simulink model "Fixed_Wing_Model"  (R2023a)
settings: Solver=FixedStepAuto  StartTime=0.0  StopTime=inf  FixedStep=model_sampling_time  RelTol=1e-3
InitFcn:
  | run("Parameters.m")
values from neighbouring files (symbols this model uses):
  Alpha = params.Aerodynamics.Alpha    [aircraft_model.m]    (also in aircraft_params.mat = [-0.698131700798 -0.680678408278 -0.663225115758 -0.64577182; cost_straight_level.m = atan2(X(3), X(1)); create_table.m = deg2rad(-40:1:40)'; nonlinear_const.m = atan2(X(3), X(1)))
  Beta = params.Aerodynamics.Beta    [aircraft_model.m]    (also in aircraft_params.mat = [-0.349065850399 -0.261799387799 -0.174532925199 -0.08726646; create_table.m = deg2rad(-20:5:20)')
  CD_alpha_beta = [0.0544509195029 0.0530405310175 0.0517292718774 0.0505171420827 0.0494041416333 0.0483902705292 0.0474755287703 0.0466599163568 0.0459434332887 0.0453260795658 0.0448078551882 0.0443887601559 ... (729 elements, 81x9)]    [aircraft_params.mat]    (also in create_table.m = zeros(length(Alpha), length(Beta)))
  CD_alpha_dot = 0    [Parameters.m]    (also in aircraft_params.mat)
  CD_u = 0    [Parameters.m]    (also in aircraft_params.mat)
  CDda = [0 0 0 0 0 0 0 0 0 0 0 0 ... (1539 elements, 19x81)]    [aircraft_params.mat]    (also in create_table.m = zeros(length(da), length(Alpha)))
  CDde = [0 0 0 0 0 0 0 0 0 0 0 0 ... (1539 elements, 19x81)]    [aircraft_params.mat]    (also in create_table.m = zeros(length(de), length(Alpha)))
  CDdr = [0 0 0 0 0 0 0 0 0 0 0 0 ... (171 elements, 19x9)]    [aircraft_params.mat]    (also in create_table.m = zeros(length(dr), length(Beta)))
  CDp = [0.00874 0.009614 0.010488 0.011362 0.012236 0.01311 0.013984 0.014858 0.015732 0.016606 0.01748 0.018354 ... (81 elements, 81x1)]    [aircraft_params.mat]    (also in create_table.m = zeros(length(Alpha),1))
  CDq = [0 0 0 0 0 0 0 0 0 0 0 0 ... (81 elements, 81x1)]    [aircraft_params.mat]    (also in create_table.m = zeros(length(Alpha),1))
  CDr = [0 0 0 0 0 0 0 0 0 0 0 0 ... (81 elements, 81x1)]    [aircraft_params.mat]    (also in create_table.m = zeros(length(Alpha),1))
  chord = 0.1894    [Parameters.m]    (also in aircraft_model.m = params.chord; aircraft_params.mat)
  CL_alpha_beta = [-0.633037607685 -0.615603980908 -0.597456739131 -0.578694538839 -0.559464427591 -0.54002303701 -0.520877191922 -0.503102694522 -0.489045924609 -0.483759795494 -0.497410215644 -0.54697394645 ... (729 elements, 81x9)]    [aircraft_params.mat]    (also in create_table.m = zeros(length(Alpha), length(Beta)))
  Cl_alpha_beta = [0.00837758040957 0.00921533845053 0.0100530964915 0.0108908545324 0.0117286125734 0.0125663706144 0.0134041286553 0.0142418866963 0.0150796447372 0.0159174027782 0.0167551608191 0.0175929188601 ... (729 elements, 81x9)]    [aircraft_params.mat]    (also in create_table.m = zeros(length(Alpha), length(Beta)))
  CL_alpha_dot = 0    [Parameters.m]    (also in aircraft_params.mat)
  Cl_alpha_dot = 0    [Parameters.m]    (also in aircraft_params.mat)
  CL_u = 0    [Parameters.m]    (also in aircraft_params.mat)
  Cl_u = 0    [Parameters.m]    (also in aircraft_params.mat)
  CLda = [0 0 0 0 0 0 0 0 0 0 0 0 ... (1539 elements, 19x81)]    [aircraft_params.mat]    (also in create_table.m = zeros(length(da), length(Alpha)))
  Clda = [-0.0125663706144 -0.0111701072128 -0.00977384381117 -0.00837758040957 -0.00698131700798 -0.00558505360638 -0.00418879020479 -0.00279252680319 -0.0013962634016 0 0.0013962634016 0.00279252680319 ... (1539 elements, 19x81)]    [aircraft_params.mat]    (also in create_table.m = zeros(length(da), length(Alpha)))
  CLde = [0.0565486677646 0.0502654824574 0.0439822971503 0.0376991118431 0.0314159265359 0.0251327412287 0.0188495559215 0.0125663706144 0.00628318530718 0 -0.00628318530718 -0.0125663706144 ... (1539 elements, 19x81)]    [aircraft_params.mat]    (also in create_table.m = zeros(length(de), length(Alpha)))
  Clde = [0 0 0 0 0 0 0 0 0 0 0 0 ... (1539 elements, 19x81)]    [aircraft_params.mat]    (also in create_table.m = zeros(length(de), length(Alpha)))
  CLdr = [0 0 0 0 0 0 0 0 0 0 0 0 ... (171 elements, 19x9)]    [aircraft_params.mat]    (also in create_table.m = zeros(length(dr), length(Beta)))
  Cldr = [-0.0758694625842 -0.0674395222971 -0.0590095820099 -0.0505796417228 -0.0421497014357 -0.0337197611485 -0.0252898208614 -0.0168598805743 -0.00842994028713 0 0.00842994028713 0.0168598805743 ... (171 elements, 19x9)]    [aircraft_params.mat]    (also in create_table.m = zeros(length(dr), length(Beta)))
  CLp = [0 0 0 0 0 0 0 0 0 0 0 0 ... (81 elements, 81x1)]    [aircraft_params.mat]    (also in create_table.m = zeros(length(Alpha),1))
  Clp = [-0.052 -0.0572 -0.0624 -0.0676 -0.0728 -0.078 -0.0832 -0.0884 -0.0936 -0.0988 -0.104 -0.1092 ... (81 elements, 81x1)]    [aircraft_params.mat]    (also in create_table.m = zeros(length(Alpha),1))
  CLq = [0 0 0 0 0 0 0 0 0 0 0 0 ... (81 elements, 81x1)]    [aircraft_params.mat]    (also in create_table.m = zeros(length(Alpha),1))
  Clq = [0 0 0 0 0 0 0 0 0 0 0 0 ... (81 elements, 81x1)]    [aircraft_params.mat]    (also in create_table.m = zeros(length(Alpha),1))
  CLr = [0 0 0 0 0 0 0 0 0 0 0 0 ... (81 elements, 81x1)]    [aircraft_params.mat]    (also in create_table.m = zeros(length(Alpha),1))
  Clr = [0.028 0.0308 0.0336 0.0364 0.0392 0.042 0.0448 0.0476 0.0504 0.0532 0.056 0.0588 ... (81 elements, 81x1)]    [aircraft_params.mat]    (also in create_table.m = zeros(length(Alpha),1))
  Cm_alpha_beta = [0.220686842599 0.214585171534 0.208483500469 0.202381829404 0.196280158339 0.190178487274 0.184076816209 0.177975145144 0.171873474079 0.165771803014 0.159670131949 0.153568460884 ... (729 elements, 81x9)]    [aircraft_params.mat]    (also in create_table.m = zeros(length(Alpha), length(Beta)))
  Cm_alpha_dot = 0    [Parameters.m]    (also in aircraft_params.mat)
  Cm_u = 0    [Parameters.m]    (also in aircraft_params.mat)
  Cmda = [0 0 0 0 0 0 0 0 0 0 0 0 ... (1539 elements, 19x81)]    [aircraft_params.mat]    (also in create_table.m = zeros(length(da), length(Alpha)))
  Cmde = [0.0785398163397 0.0698131700798 0.0610865238198 0.0523598775598 0.0436332312999 0.0349065850399 0.0261799387799 0.0174532925199 0.00872664625997 0 -0.00872664625997 -0.0174532925199 ... (1539 elements, 19x81)]    [aircraft_params.mat]    (also in create_table.m = zeros(length(de), length(Alpha)))
  Cmdr = [0 0 0 0 0 0 0 0 0 0 0 0 ... (171 elements, 19x9)]    [aircraft_params.mat]    (also in create_table.m = zeros(length(dr), length(Beta)))
  Cmp = [0 0 0 0 0 0 0 0 0 0 0 0 ... (81 elements, 81x1)]    [aircraft_params.mat]    (also in create_table.m = zeros(length(Alpha),1))
  Cmq = [-0.72 -0.792 -0.864 -0.936 -1.008 -1.08 -1.152 -1.224 -1.296 -1.368 -1.44 -1.512 ... (81 elements, 81x1)]    [aircraft_params.mat]    (also in create_table.m = zeros(length(Alpha),1))
  Cmr = [0 0 0 0 0 0 0 0 0 0 0 0 ... (81 elements, 81x1)]    [aircraft_params.mat]    (also in create_table.m = zeros(length(Alpha),1))
  Cn_alpha_beta = [-0.0174532925199 -0.0191986217719 -0.0209439510239 -0.0226892802759 -0.0244346095279 -0.0261799387799 -0.0279252680319 -0.0296705972839 -0.0314159265359 -0.0331612557879 -0.0349065850399 -0.0366519142919 ... (729 elements, 81x9)]    [aircraft_params.mat]    (also in create_table.m = zeros(length(Alpha), length(Beta)))
  Cn_alpha_dot = 0    [Parameters.m]    (also in aircraft_params.mat)
  Cn_u = 0    [Parameters.m]    (also in aircraft_params.mat)
  Cnda = [-0.00942477796077 -0.00837758040957 -0.00733038285838 -0.00628318530718 -0.00523598775598 -0.00418879020479 -0.00314159265359 -0.00209439510239 -0.0010471975512 0 0.0010471975512 0.00209439510239 ... (1539 elements, 19x81)]    [aircraft_params.mat]    (also in create_table.m = zeros(length(da), length(Alpha)))
  Cnde = [0 0 0 0 0 0 0 0 0 0 0 0 ... (1539 elements, 19x81)]    [aircraft_params.mat]    (also in create_table.m = zeros(length(de), length(Alpha)))
  Cndr = [0.0231221219304 0.0205529972715 0.0179838726125 0.0154147479536 0.0128456232947 0.0102764986357 0.00770737397681 0.00513824931787 0.00256912465894 0 -0.00256912465894 -0.00513824931787 ... (171 elements, 19x9)]    [aircraft_params.mat]    (also in create_table.m = zeros(length(dr), length(Beta)))
  Cnp = [0.0044 0.00484 0.00528 0.00572 0.00616 0.0066 0.00704 0.00748 0.00792 0.00836 0.0088 0.00924 ... (81 elements, 81x1)]    [aircraft_params.mat]    (also in create_table.m = zeros(length(Alpha),1))
  Cnq = [0 0 0 0 0 0 0 0 0 0 0 0 ... (81 elements, 81x1)]    [aircraft_params.mat]    (also in create_table.m = zeros(length(Alpha),1))
  Cnr = [-0.07 -0.077 -0.084 -0.091 -0.098 -0.105 -0.112 -0.119 -0.126 -0.133 -0.14 -0.147 ... (81 elements, 81x1)]    [aircraft_params.mat]    (also in create_table.m = zeros(length(Alpha),1))
  CY_alpha_beta = [0.0684169066782 0.075258597346 0.0821002880138 0.0889419786816 0.0957836693494 0.102625360017 0.109467050685 0.116308741353 0.123150432021 0.129992122689 0.136833813356 0.143675504024 ... (729 elements, 81x9)]    [aircraft_params.mat]    (also in create_table.m = zeros(length(Alpha), length(Beta)))
  CY_alpha_dot = 0    [Parameters.m]    (also in aircraft_params.mat)
  CY_u = 0    [Parameters.m]    (also in aircraft_params.mat)
  CYda = [0 0 0 0 0 0 0 0 0 0 0 0 ... (1539 elements, 19x81)]    [aircraft_params.mat]    (also in create_table.m = zeros(length(da), length(Alpha)))
  CYde = [0 0 0 0 0 0 0 0 0 0 0 0 ... (1539 elements, 19x81)]    [aircraft_params.mat]    (also in create_table.m = zeros(length(de), length(Alpha)))
  CYdr = [0.122836272755 0.109187798005 0.0955393232542 0.0818908485036 0.068242373753 0.0545938990024 0.0409454242518 0.0272969495012 0.0136484747506 0 -0.0136484747506 -0.0272969495012 ... (171 elements, 19x9)]    [aircraft_params.mat]    (also in create_table.m = zeros(length(dr), length(Beta)))
  CYp = [0 0 0 0 0 0 0 0 0 0 0 0 ... (81 elements, 81x1)]    [aircraft_params.mat]    (also in create_table.m = zeros(length(Alpha),1))
  CYq = [0 0 0 0 0 0 0 0 0 0 0 0 ... (81 elements, 81x1)]    [aircraft_params.mat]    (also in create_table.m = zeros(length(Alpha),1))
  CYr = [0 0 0 0 0 0 0 0 0 0 0 0 ... (81 elements, 81x1)]    [aircraft_params.mat]    (also in create_table.m = zeros(length(Alpha),1))
  D = zeros(size(B_long))    [Linearized_Model.m]    (also in linear_models.mat = [0 0 0 0 0 0 0 0 0 0 0 0 ... (16 elements, 4x4)])
  da = params.Aerodynamics.da    [aircraft_model.m]    (also in aircraft_params.mat = [-0.785398163397 -0.698131700798 -0.610865238198 -0.52359877; create_table.m = deg2rad(-45:5:45))
  da_lim = deg2rad(45)    [Parameters.m]    (also in aircraft_model.m = params.da_lim; aircraft_params.mat = 0.785398163397)
  de_lim = deg2rad(45)    [Parameters.m]    (also in aircraft_model.m = params.de_lim; aircraft_params.mat = 0.785398163397)
  dr = params.Aerodynamics.dr    [aircraft_model.m]    (also in aircraft_params.mat = [-0.785398163397 -0.698131700798 -0.610865238198 -0.52359877; create_table.m = deg2rad(-45:5:45))
  dr_lim = deg2rad(45)    [Parameters.m]    (also in aircraft_model.m = params.dr_lim; aircraft_params.mat = 0.785398163397)
  dth_lim = 100    [Parameters.m]    (also in aircraft_model.m = params.dth_lim; aircraft_params.mat)
  h_ref = 0    [Parameters.m]    (also in aircraft_params.mat)
  Inertia_Tensor = [Jx -Jxy -Jxz ... (first row only)    [Parameters.m]    (also in aircraft_model.m; aircraft_params.mat = [0.8244  0  -0.1204; 0  1.135  0; -0.1204  0  1.759])
  lat_ref_deg = 40    [Parameters.m]    (also in aircraft_params.mat)
  long_ref_deg = 20    [Parameters.m]    (also in aircraft_params.mat)
  mass = 13.5    [Parameters.m]    (also in aircraft_model.m = params.mass; aircraft_params.mat)
  Motor =     [aircraft_params.mat]
  pqr_initial = [0; 0; 0]    [Parameters.m]    (also in aircraft_params.mat = [0 0 0])
  quat_initial = eul2quat(euler_initial')    [Parameters.m]    (also in aircraft_params.mat = [1 0 0 0])
  rho_msl = 1.225    [Parameters.m]    (also in aircraft_model.m = params.rho_msl; aircraft_params.mat)
  S = 2.8956    [Parameters.m]    (also in aircraft_model.m = params.S; aircraft_params.mat)
  v_body_initial = [30; 0; 0]    [Parameters.m]    (also in aircraft_params.mat = [30 0 0])
  wing_span = 0.55    [Parameters.m]    (also in aircraft_model.m = params.wing_span; aircraft_params.mat)
undefined symbols (not defined in the file or in its folder): DiscIntNeverNeededParam, Earth, lat_deg, long_deg, WGS84
libraries: simulink x20, aerolibutil x5, matrix_library x2, aerolibtransform2 x2, sharedtransform x2, simulink_extras x2, sharedutil x1, aerolibatmos2 x1, aerolibsim3d x1, sim3dlib x1
(part 2 of 2)

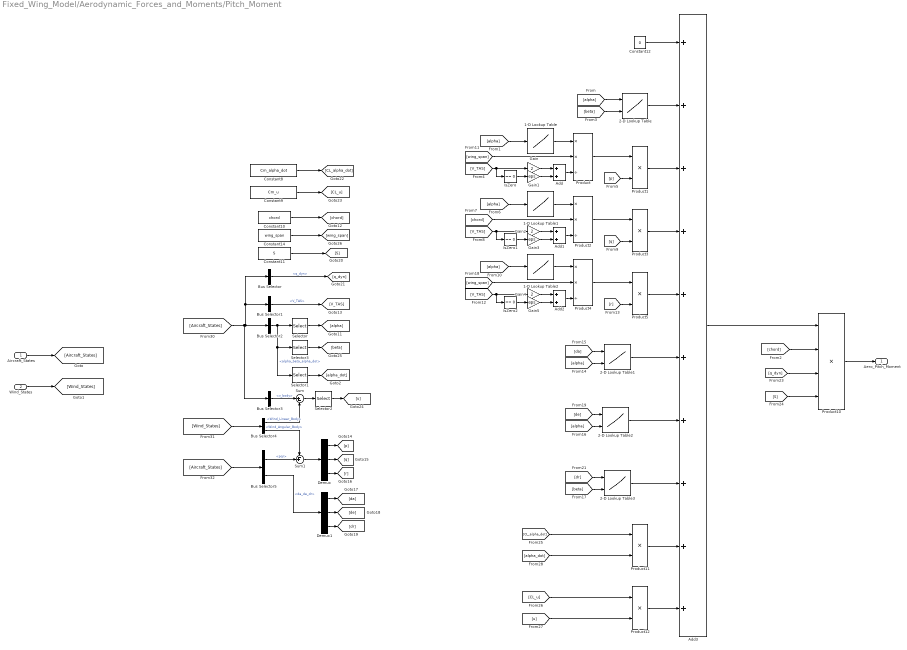
== system Fixed_Wing_Model/Aerodynamic_Forces_and_Moments/Pitch_Moment ==
  Aircraft_States : Inport
  Wind_States : Inport  Port=2
  1-D Lookup Table : Lookup_n-D  NumberOfTableDimensions=1  BreakpointsForDimension1=Alpha  Table=Cmp  InternalRulePriority=Speed  RndMeth=Simplest
  1-D Lookup Table1 : Lookup_n-D  NumberOfTableDimensions=1  BreakpointsForDimension1=Alpha  Table=Cmq  InternalRulePriority=Speed  RndMeth=Simplest
  1-D Lookup Table2 : Lookup_n-D  NumberOfTableDimensions=1  BreakpointsForDimension1=Alpha  Table=Cmr  InternalRulePriority=Speed  RndMeth=Simplest
  2-D Lookup Table : Lookup_n-D  BreakpointsForDimension1=Alpha  BreakpointsForDimension2=Beta  Table=Cm_alpha_beta  InternalRulePriority=Speed  RndMeth=Simplest
      settings: InputPortMap=u0,u1
  2-D Lookup Table1 : Lookup_n-D  BreakpointsForDimension1=da  BreakpointsForDimension2=Alpha  Table=Cmda  InternalRulePriority=Speed  RndMeth=Simplest
      settings: InputPortMap=u0,u1
  2-D Lookup Table2 : Lookup_n-D  BreakpointsForDimension1=da  BreakpointsForDimension2=Alpha  Table=Cmde  InternalRulePriority=Speed  RndMeth=Simplest
      settings: InputPortMap=u0,u1
  2-D Lookup Table3 : Lookup_n-D  BreakpointsForDimension1=dr  BreakpointsForDimension2=Beta  Table=Cmdr  InternalRulePriority=Speed  RndMeth=Simplest
      settings: InputPortMap=u0,u1
  Add : Sum
  Add1 : Sum
  Add2 : Sum
  Add3 : Sum  Inputs=10
  Bus Selector : BusSelector  OutputSignals=q_dyn
  Bus Selector1 : BusSelector  OutputSignals=V_TAS
  Bus Selector2 : BusSelector  OutputSignals=alpha_beta_alpha_dot
  Bus Selector3 : BusSelector  OutputSignals=v_body
  Bus Selector4 : BusSelector  OutputSignals=Wind_Linear_Body,Wind_Angular_Body
  Bus Selector5 : BusSelector  OutputSignals=pqr,da_de_dr
  Constant10 : Constant  Value=chord
  Constant11 : Constant  Value=S
  Constant12 : Constant  Value=0
  Constant14 : Constant  Value=wing_span
  Constant8 : Constant  Value=Cm_alpha_dot
  Constant9 : Constant  Value=Cm_u
  Demux : Demux  Outputs=3
  Demux1 : Demux  Outputs=3
  Gain : Gain  Gain=2
  Gain1 : Gain  Gain=eps
  Gain2 : Gain  Gain=2
  Gain3 : Gain  Gain=eps
  Gain4 : Gain  Gain=2
  Gain5 : Gain  Gain=eps
  IsZero : simulink/Logic and Bit Operations/Compare To Zero  relop===  OutDataTypeStr=uint8
      settings: LibrarySourceBlock=|
      | simulink/Quick Insert/Logic and Bit
      | Operations/IsZero
  IsZero1 : simulink/Logic and Bit Operations/Compare To Zero  relop===  OutDataTypeStr=uint8
      settings: LibrarySourceBlock=|
      | simulink/Quick Insert/Logic and Bit
      | Operations/IsZero
  IsZero2 : simulink/Logic and Bit Operations/Compare To Zero  relop===  OutDataTypeStr=uint8
      settings: LibrarySourceBlock=|
      | simulink/Quick Insert/Logic and Bit
      | Operations/IsZero
  Product : Product  Inputs=**/
  Product{1,3,5,11..12} (5 alike) : Product
  Product10 : Product  Inputs=4
  Product2 : Product  Inputs=**/
  Product4 : Product  Inputs=**/
  Selector : Selector  InputPortWidth=3  IndexOptions=Index vector (dialog)  Indices=1  OutputSizes=1
  Selector1 : Selector  InputPortWidth=3  IndexOptions=Index vector (dialog)  Indices=3  OutputSizes=1
  Selector2 : Selector  InputPortWidth=3  IndexOptions=Index vector (dialog)  Indices=1  OutputSizes=1
  Selector3 : Selector  InputPortWidth=3  IndexOptions=Index vector (dialog)  Indices=2  OutputSizes=1
  Sum : Sum  Inputs=|+-
  Sum1 : Sum  Inputs=-+|
  Aero_Pitch_Moment : Outport  Unit=N*m
  wires:
  Constant14/1 -> [wing_span]
  [beta] -> 2-D Lookup Table3/2
  [dr] -> 2-D Lookup Table3/1
  [alpha] -> 2-D Lookup Table2/2
  [da] -> 2-D Lookup Table1/1
  [alpha] -> 2-D Lookup Table1/2
  [alpha] -> 1-D Lookup Table2/1
  1-D Lookup Table2/1 -> Product4/1
  [alpha] -> 1-D Lookup Table1/1
  1-D Lookup Table1/1 -> Product2/1
  [alpha] -> 1-D Lookup Table/1
  1-D Lookup Table/1 -> Product/1
  [beta] -> 2-D Lookup Table/2
  [alpha] -> 2-D Lookup Table/1
  Selector3/1 -> [beta]
  Bus Selector5/2 -> Demux1/1  "<da_de_dr>"
  Bus Selector5/1 -> Sum1/2  "<pqr>"
  [Aircraft_States] -> Bus Selector5/1
  Bus Selector4/2 -> Sum1/1  "<Wind_Angular_Body>"
  Sum1/1 -> Demux/1
  Sum/1 -> Selector2/1
  Bus Selector3/1 -> Sum/1  "<v_body>"
  Bus Selector4/1 -> Sum/2  "<Wind_Linear_Body>"
  [Wind_States] -> Bus Selector4/1
  Selector2/1 -> [u]
  Selector1/1 -> [alpha_dot]
  Selector/1 -> [alpha]
  Bus Selector2/1 -> Selector/1, Selector1/1, Selector3/1  "<alpha_beta_alpha_dot>"
  Bus Selector1/1 -> [V_TAS]  "<V_TAS>"
  Bus Selector/1 -> [q_dyn]  "<q_dyn>"
  [Aircraft_States] -> Bus Selector2/1, Bus Selector1/1, Bus Selector/1, Bus Selector3/1
  Wind_States/1 -> [Wind_States]
  Aircraft_States/1 -> [Aircraft_States]
  Demux1/3 -> [dr]
  2-D Lookup Table2/1 -> Add3/7
  [S] -> Product10/4
  Gain1/1 -> Add/2
  [V_TAS] -> IsZero2/1, Gain4/1
  [V_TAS] -> IsZero/1, Gain/1
  Add2/1 -> Product4/3
  Add/1 -> Product/3
  Constant12/1 -> Add3/1
  Product2/1 -> Product3/1
  [chord] -> Product10/2
  Add1/1 -> Product2/3
  Gain5/1 -> Add2/2
  Product4/1 -> Product5/1
  2-D Lookup Table1/1 -> Add3/6
  [q] -> Product3/2
  Add3/1 -> Product10/1
  Demux/3 -> [r]
  [V_TAS] -> Gain2/1, IsZero1/1
  Product5/1 -> Add3/5
  Gain/1 -> Add/1
  Gain4/1 -> Add2/1
  Gain3/1 -> Add1/2
  IsZero2/1 -> Gain5/1
  Gain2/1 -> Add1/1
  [q_dyn] -> Product10/3
  Demux1/1 -> [da]
  [chord] -> Product2/2
  IsZero1/1 -> Gain3/1
  [r] -> Product5/2
  [wing_span] -> Product/2
  Product/1 -> Product1/1
  Product1/1 -> Add3/3
  [p] -> Product1/2
  IsZero/1 -> Gain1/1
  2-D Lookup Table/1 -> Add3/2
  [wing_span] -> Product4/2
  Product3/1 -> Add3/4
  [de] -> 2-D Lookup Table2/1
  2-D Lookup Table3/1 -> Add3/8
  Demux/2 -> [q]
  Demux1/2 -> [de]
  Demux/1 -> [p]
  Product10/1 -> Aero_Pitch_Moment/1
  Constant10/1 -> [chord]
  Constant8/1 -> [CL_alpha_dot]
  Constant9/1 -> [CL_u]
  Constant11/1 -> [S]
  Product11/1 -> Add3/9
  [CL_alpha_dot] -> Product11/1
  Product12/1 -> Add3/10
  [CL_u] -> Product12/1
  [alpha_dot] -> Product11/2
  [u] -> Product12/2

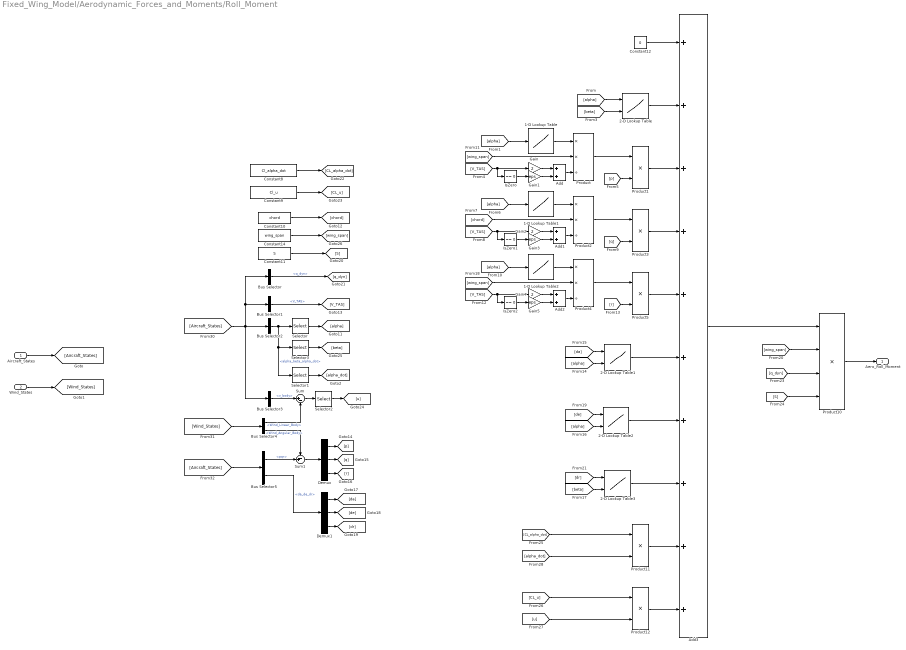
== system Fixed_Wing_Model/Aerodynamic_Forces_and_Moments/Roll_Moment ==
  Aircraft_States : Inport
  Wind_States : Inport  Port=2
  1-D Lookup Table : Lookup_n-D  NumberOfTableDimensions=1  BreakpointsForDimension1=Alpha  Table=Clp  InternalRulePriority=Speed  RndMeth=Simplest
  1-D Lookup Table1 : Lookup_n-D  NumberOfTableDimensions=1  BreakpointsForDimension1=Alpha  Table=Clq  InternalRulePriority=Speed  RndMeth=Simplest
  1-D Lookup Table2 : Lookup_n-D  NumberOfTableDimensions=1  BreakpointsForDimension1=Alpha  Table=Clr  InternalRulePriority=Speed  RndMeth=Simplest
  2-D Lookup Table : Lookup_n-D  BreakpointsForDimension1=Alpha  BreakpointsForDimension2=Beta  Table=Cl_alpha_beta  InternalRulePriority=Speed  RndMeth=Simplest
      settings: InputPortMap=u0,u1
  2-D Lookup Table1 : Lookup_n-D  BreakpointsForDimension1=da  BreakpointsForDimension2=Alpha  Table=Clda  InternalRulePriority=Speed  RndMeth=Simplest
      settings: InputPortMap=u0,u1
  2-D Lookup Table2 : Lookup_n-D  BreakpointsForDimension1=da  BreakpointsForDimension2=Alpha  Table=Clde  InternalRulePriority=Speed  RndMeth=Simplest
      settings: InputPortMap=u0,u1
  2-D Lookup Table3 : Lookup_n-D  BreakpointsForDimension1=dr  BreakpointsForDimension2=Beta  Table=Cldr  InternalRulePriority=Speed  RndMeth=Simplest
      settings: InputPortMap=u0,u1
  Add : Sum
  Add1 : Sum
  Add2 : Sum
  Add3 : Sum  Inputs=10
  Bus Selector : BusSelector  OutputSignals=q_dyn
  Bus Selector1 : BusSelector  OutputSignals=V_TAS
  Bus Selector2 : BusSelector  OutputSignals=alpha_beta_alpha_dot
  Bus Selector3 : BusSelector  OutputSignals=v_body
  Bus Selector4 : BusSelector  OutputSignals=Wind_Linear_Body,Wind_Angular_Body
  Bus Selector5 : BusSelector  OutputSignals=pqr,da_de_dr
  Constant10 : Constant  Value=chord
  Constant11 : Constant  Value=S
  Constant12 : Constant  Value=0
  Constant14 : Constant  Value=wing_span
  Constant8 : Constant  Value=Cl_alpha_dot
  Constant9 : Constant  Value=Cl_u
  Demux : Demux  Outputs=3
  Demux1 : Demux  Outputs=3
  Gain : Gain  Gain=2
  Gain1 : Gain  Gain=eps
  Gain2 : Gain  Gain=2
  Gain3 : Gain  Gain=eps
  Gain4 : Gain  Gain=2
  Gain5 : Gain  Gain=eps
  IsZero : simulink/Logic and Bit Operations/Compare To Zero  relop===  OutDataTypeStr=uint8
      settings: LibrarySourceBlock=|
      | simulink/Quick Insert/Logic and Bit
      | Operations/IsZero
  IsZero1 : simulink/Logic and Bit Operations/Compare To Zero  relop===  OutDataTypeStr=uint8
      settings: LibrarySourceBlock=|
      | simulink/Quick Insert/Logic and Bit
      | Operations/IsZero
  IsZero2 : simulink/Logic and Bit Operations/Compare To Zero  relop===  OutDataTypeStr=uint8
      settings: LibrarySourceBlock=|
      | simulink/Quick Insert/Logic and Bit
      | Operations/IsZero
  Product : Product  Inputs=**/
  Product{1,3,5,11..12} (5 alike) : Product
  Product10 : Product  Inputs=4
  Product2 : Product  Inputs=**/
  Product4 : Product  Inputs=**/
  Selector : Selector  InputPortWidth=3  IndexOptions=Index vector (dialog)  Indices=1  OutputSizes=1
  Selector1 : Selector  InputPortWidth=3  IndexOptions=Index vector (dialog)  Indices=3  OutputSizes=1
  Selector2 : Selector  InputPortWidth=3  IndexOptions=Index vector (dialog)  Indices=1  OutputSizes=1
  Selector3 : Selector  InputPortWidth=3  IndexOptions=Index vector (dialog)  Indices=2  OutputSizes=1
  Sum : Sum  Inputs=|+-
  Sum1 : Sum  Inputs=-+|
  Aero_Roll_Moment : Outport  Unit=N*m
  wires:
  [u] -> Product12/2
  [alpha_dot] -> Product11/2
  [CL_u] -> Product12/1
  Product12/1 -> Add3/10
  [CL_alpha_dot] -> Product11/1
  Product11/1 -> Add3/9
  Constant11/1 -> [S]
  Constant9/1 -> [CL_u]
  Constant8/1 -> [CL_alpha_dot]
  Constant10/1 -> [chord]
  Product10/1 -> Aero_Roll_Moment/1
  Demux/1 -> [p]
  Demux1/2 -> [de]
  Demux/2 -> [q]
  2-D Lookup Table3/1 -> Add3/8
  [de] -> 2-D Lookup Table2/1
  Product3/1 -> Add3/4
  [wing_span] -> Product4/2
  2-D Lookup Table/1 -> Add3/2
  IsZero/1 -> Gain1/1
  [p] -> Product1/2
  Product1/1 -> Add3/3
  Product/1 -> Product1/1
  [wing_span] -> Product/2
  [r] -> Product5/2
  IsZero1/1 -> Gain3/1
  [chord] -> Product2/2
  Demux1/1 -> [da]
  [q_dyn] -> Product10/3
  Gain2/1 -> Add1/1
  IsZero2/1 -> Gain5/1
  Gain3/1 -> Add1/2
  Gain4/1 -> Add2/1
  Gain/1 -> Add/1
  Product5/1 -> Add3/5
  [V_TAS] -> IsZero1/1, Gain2/1
  Demux/3 -> [r]
  Add3/1 -> Product10/1
  [q] -> Product3/2
  2-D Lookup Table1/1 -> Add3/6
  Product4/1 -> Product5/1
  Gain5/1 -> Add2/2
  Add1/1 -> Product2/3
  [wing_span] -> Product10/2
  Product2/1 -> Product3/1
  Constant12/1 -> Add3/1
  Add/1 -> Product/3
  Add2/1 -> Product4/3
  [V_TAS] -> Gain/1, IsZero/1
  [V_TAS] -> Gain4/1, IsZero2/1
  Gain1/1 -> Add/2
  [S] -> Product10/4
  2-D Lookup Table2/1 -> Add3/7
  Demux1/3 -> [dr]
  Aircraft_States/1 -> [Aircraft_States]
  Wind_States/1 -> [Wind_States]
  [Aircraft_States] -> Bus Selector3/1, Bus Selector/1, Bus Selector1/1, Bus Selector2/1
  Bus Selector/1 -> [q_dyn]  "<q_dyn>"
  Bus Selector1/1 -> [V_TAS]  "<V_TAS>"
  Bus Selector2/1 -> Selector3/1, Selector1/1, Selector/1  "<alpha_beta_alpha_dot>"
  Selector/1 -> [alpha]
  Selector1/1 -> [alpha_dot]
  Selector2/1 -> [u]
  [Wind_States] -> Bus Selector4/1
  Bus Selector4/1 -> Sum/2  "<Wind_Linear_Body>"
  Bus Selector3/1 -> Sum/1  "<v_body>"
  Sum/1 -> Selector2/1
  Sum1/1 -> Demux/1
  Bus Selector4/2 -> Sum1/1  "<Wind_Angular_Body>"
  [Aircraft_States] -> Bus Selector5/1
  Bus Selector5/1 -> Sum1/2  "<pqr>"
  Bus Selector5/2 -> Demux1/1  "<da_de_dr>"
  Selector3/1 -> [beta]
  [alpha] -> 2-D Lookup Table/1
  [beta] -> 2-D Lookup Table/2
  1-D Lookup Table/1 -> Product/1
  [alpha] -> 1-D Lookup Table/1
  1-D Lookup Table1/1 -> Product2/1
  [alpha] -> 1-D Lookup Table1/1
  1-D Lookup Table2/1 -> Product4/1
  [alpha] -> 1-D Lookup Table2/1
  [alpha] -> 2-D Lookup Table1/2
  [da] -> 2-D Lookup Table1/1
  [alpha] -> 2-D Lookup Table2/2
  [dr] -> 2-D Lookup Table3/1
  [beta] -> 2-D Lookup Table3/2
  Constant14/1 -> [wing_span]

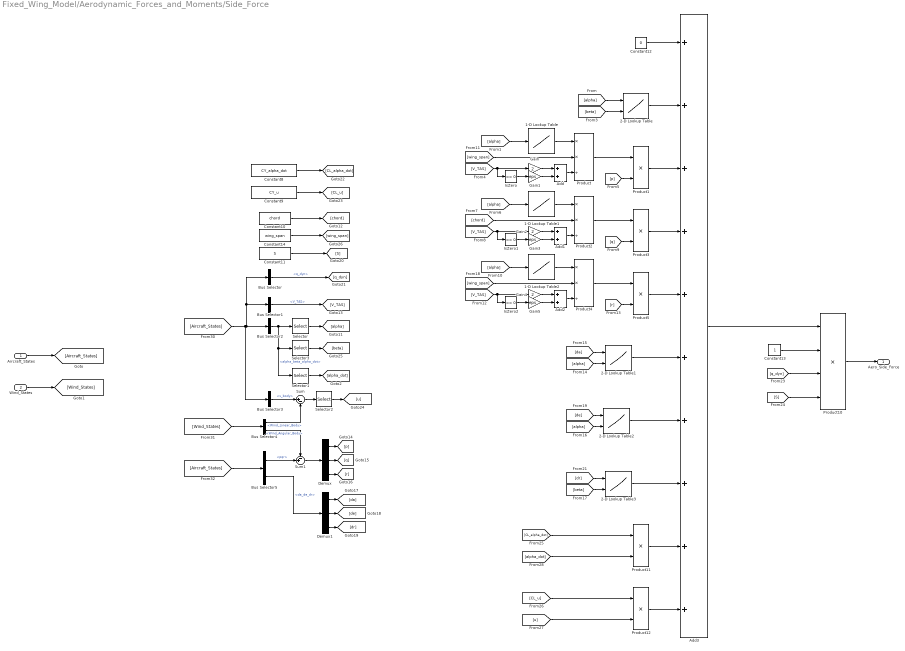
== system Fixed_Wing_Model/Aerodynamic_Forces_and_Moments/Side_Force ==
  Aircraft_States : Inport
  Wind_States : Inport  Port=2
  1-D Lookup Table : Lookup_n-D  NumberOfTableDimensions=1  BreakpointsForDimension1=Alpha  Table=CYp  InternalRulePriority=Speed  RndMeth=Simplest
  1-D Lookup Table1 : Lookup_n-D  NumberOfTableDimensions=1  BreakpointsForDimension1=Alpha  Table=CYq  InternalRulePriority=Speed  RndMeth=Simplest
  1-D Lookup Table2 : Lookup_n-D  NumberOfTableDimensions=1  BreakpointsForDimension1=Alpha  Table=CYr  InternalRulePriority=Speed  RndMeth=Simplest
  2-D Lookup Table : Lookup_n-D  BreakpointsForDimension1=Alpha  BreakpointsForDimension2=Beta  Table=CY_alpha_beta  InternalRulePriority=Speed  RndMeth=Simplest
      settings: InputPortMap=u0,u1
  2-D Lookup Table1 : Lookup_n-D  BreakpointsForDimension1=da  BreakpointsForDimension2=Alpha  Table=CYda  InternalRulePriority=Speed  RndMeth=Simplest
      settings: InputPortMap=u0,u1
  2-D Lookup Table2 : Lookup_n-D  BreakpointsForDimension1=da  BreakpointsForDimension2=Alpha  Table=CYde  InternalRulePriority=Speed  RndMeth=Simplest
      settings: InputPortMap=u0,u1
  2-D Lookup Table3 : Lookup_n-D  BreakpointsForDimension1=dr  BreakpointsForDimension2=Beta  Table=CYdr  InternalRulePriority=Speed  RndMeth=Simplest
      settings: InputPortMap=u0,u1
  Add : Sum
  Add1 : Sum
  Add2 : Sum
  Add3 : Sum  Inputs=10
  Bus Selector : BusSelector  OutputSignals=q_dyn
  Bus Selector1 : BusSelector  OutputSignals=V_TAS
  Bus Selector2 : BusSelector  OutputSignals=alpha_beta_alpha_dot
  Bus Selector3 : BusSelector  OutputSignals=v_body
  Bus Selector4 : BusSelector  OutputSignals=Wind_Linear_Body,Wind_Angular_Body
  Bus Selector5 : BusSelector  OutputSignals=pqr,da_de_dr
  Constant10 : Constant  Value=chord
  Constant11 : Constant  Value=S
  Constant12 : Constant  Value=0
  Constant13 : Constant
  Constant14 : Constant  Value=wing_span
  Constant8 : Constant  Value=CY_alpha_dot
  Constant9 : Constant  Value=CY_u
  Demux : Demux  Outputs=3
  Demux1 : Demux  Outputs=3
  Gain : Gain  Gain=2
  Gain1 : Gain  Gain=eps
  Gain2 : Gain  Gain=2
  Gain3 : Gain  Gain=eps
  Gain4 : Gain  Gain=2
  Gain5 : Gain  Gain=eps
  IsZero : simulink/Logic and Bit Operations/Compare To Zero  relop===  OutDataTypeStr=uint8
      settings: LibrarySourceBlock=|
      | simulink/Quick Insert/Logic and Bit
      | Operations/IsZero
  IsZero1 : simulink/Logic and Bit Operations/Compare To Zero  relop===  OutDataTypeStr=uint8
      settings: LibrarySourceBlock=|
      | simulink/Quick Insert/Logic and Bit
      | Operations/IsZero
  IsZero2 : simulink/Logic and Bit Operations/Compare To Zero  relop===  OutDataTypeStr=uint8
      settings: LibrarySourceBlock=|
      | simulink/Quick Insert/Logic and Bit
      | Operations/IsZero
  Product : Product  Inputs=**/
  Product{1,3,5,11..12} (5 alike) : Product
  Product10 : Product  Inputs=4
  Product2 : Product  Inputs=**/
  Product4 : Product  Inputs=**/
  Selector : Selector  InputPortWidth=3  IndexOptions=Index vector (dialog)  Indices=1  OutputSizes=1
  Selector1 : Selector  InputPortWidth=3  IndexOptions=Index vector (dialog)  Indices=3  OutputSizes=1
  Selector2 : Selector  InputPortWidth=3  IndexOptions=Index vector (dialog)  Indices=1  OutputSizes=1
  Selector3 : Selector  InputPortWidth=3  IndexOptions=Index vector (dialog)  Indices=2  OutputSizes=1
  Sum : Sum  Inputs=|+-
  Sum1 : Sum  Inputs=-+|
  Aero_Side_Force : Outport  Unit=N*m
  wires:
  [u] -> Product12/2
  [alpha_dot] -> Product11/2
  [CL_u] -> Product12/1
  Product12/1 -> Add3/10
  [CL_alpha_dot] -> Product11/1
  Product11/1 -> Add3/9
  Constant11/1 -> [S]
  Constant9/1 -> [CL_u]
  Constant8/1 -> [CL_alpha_dot]
  Constant10/1 -> [chord]
  Product10/1 -> Aero_Side_Force/1
  Demux/1 -> [p]
  Demux1/2 -> [de]
  Demux/2 -> [q]
  2-D Lookup Table3/1 -> Add3/8
  [de] -> 2-D Lookup Table2/1
  Product3/1 -> Add3/4
  [wing_span] -> Product4/2
  2-D Lookup Table/1 -> Add3/2
  IsZero/1 -> Gain1/1
  [p] -> Product1/2
  Product1/1 -> Add3/3
  Product/1 -> Product1/1
  [wing_span] -> Product/2
  [r] -> Product5/2
  IsZero1/1 -> Gain3/1
  [chord] -> Product2/2
  Demux1/1 -> [da]
  [q_dyn] -> Product10/3
  Gain2/1 -> Add1/1
  IsZero2/1 -> Gain5/1
  Gain3/1 -> Add1/2
  Gain4/1 -> Add2/1
  Gain/1 -> Add/1
  Product5/1 -> Add3/5
  [V_TAS] -> IsZero1/1, Gain2/1
  Demux/3 -> [r]
  Add3/1 -> Product10/1
  [q] -> Product3/2
  2-D Lookup Table1/1 -> Add3/6
  Product4/1 -> Product5/1
  Gain5/1 -> Add2/2
  Add1/1 -> Product2/3
  Constant13/1 -> Product10/2
  Product2/1 -> Product3/1
  Constant12/1 -> Add3/1
  Add/1 -> Product/3
  Add2/1 -> Product4/3
  [V_TAS] -> Gain/1, IsZero/1
  [V_TAS] -> Gain4/1, IsZero2/1
  Gain1/1 -> Add/2
  [S] -> Product10/4
  2-D Lookup Table2/1 -> Add3/7
  Demux1/3 -> [dr]
  Aircraft_States/1 -> [Aircraft_States]
  Wind_States/1 -> [Wind_States]
  [Aircraft_States] -> Bus Selector3/1, Bus Selector/1, Bus Selector1/1, Bus Selector2/1
  Bus Selector/1 -> [q_dyn]  "<q_dyn>"
  Bus Selector1/1 -> [V_TAS]  "<V_TAS>"
  Bus Selector2/1 -> Selector3/1, Selector1/1, Selector/1  "<alpha_beta_alpha_dot>"
  Selector/1 -> [alpha]
  Selector1/1 -> [alpha_dot]
  Selector2/1 -> [u]
  [Wind_States] -> Bus Selector4/1
  Bus Selector4/1 -> Sum/2  "<Wind_Linear_Body>"
  Bus Selector3/1 -> Sum/1  "<v_body>"
  Sum/1 -> Selector2/1
  Sum1/1 -> Demux/1
  Bus Selector4/2 -> Sum1/1  "<Wind_Angular_Body>"
  [Aircraft_States] -> Bus Selector5/1
  Bus Selector5/1 -> Sum1/2  "<pqr>"
  Bus Selector5/2 -> Demux1/1  "<da_de_dr>"
  Selector3/1 -> [beta]
  [alpha] -> 2-D Lookup Table/1
  [beta] -> 2-D Lookup Table/2
  1-D Lookup Table/1 -> Product/1
  [alpha] -> 1-D Lookup Table/1
  1-D Lookup Table1/1 -> Product2/1
  [alpha] -> 1-D Lookup Table1/1
  1-D Lookup Table2/1 -> Product4/1
  [alpha] -> 1-D Lookup Table2/1
  [alpha] -> 2-D Lookup Table1/2
  [da] -> 2-D Lookup Table1/1
  [alpha] -> 2-D Lookup Table2/2
  [dr] -> 2-D Lookup Table3/1
  [beta] -> 2-D Lookup Table3/2
  Constant14/1 -> [wing_span]

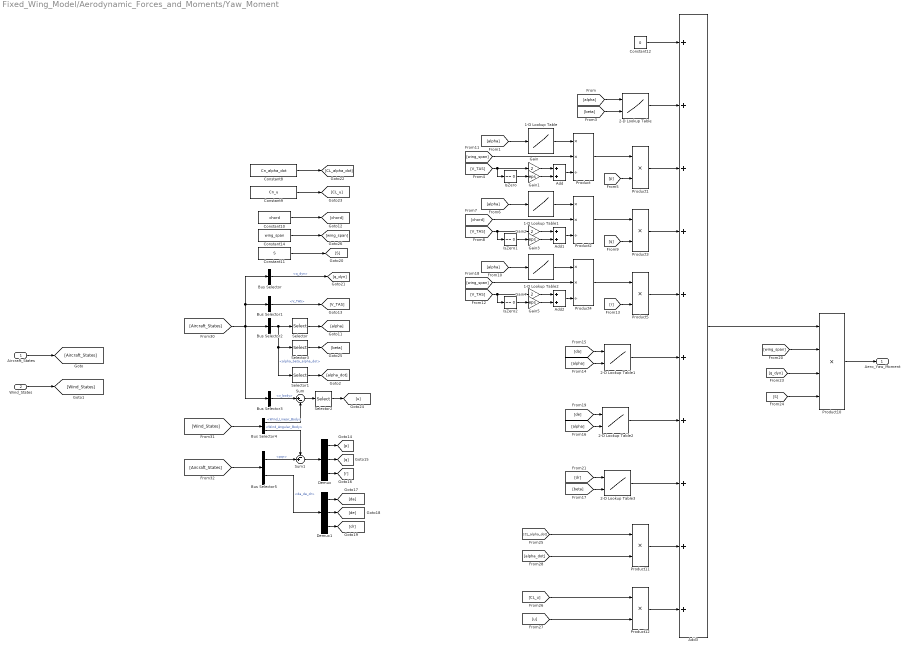
== system Fixed_Wing_Model/Aerodynamic_Forces_and_Moments/Yaw_Moment ==
  Aircraft_States : Inport
  Wind_States : Inport  Port=2
  1-D Lookup Table : Lookup_n-D  NumberOfTableDimensions=1  BreakpointsForDimension1=Alpha  Table=Cnp  InternalRulePriority=Speed  RndMeth=Simplest
  1-D Lookup Table1 : Lookup_n-D  NumberOfTableDimensions=1  BreakpointsForDimension1=Alpha  Table=Cnq  InternalRulePriority=Speed  RndMeth=Simplest
  1-D Lookup Table2 : Lookup_n-D  NumberOfTableDimensions=1  BreakpointsForDimension1=Alpha  Table=Cnr  InternalRulePriority=Speed  RndMeth=Simplest
  2-D Lookup Table : Lookup_n-D  BreakpointsForDimension1=Alpha  BreakpointsForDimension2=Beta  Table=Cn_alpha_beta  InternalRulePriority=Speed  RndMeth=Simplest
      settings: InputPortMap=u0,u1
  2-D Lookup Table1 : Lookup_n-D  BreakpointsForDimension1=da  BreakpointsForDimension2=Alpha  Table=Cnda  InternalRulePriority=Speed  RndMeth=Simplest
      settings: InputPortMap=u0,u1
  2-D Lookup Table2 : Lookup_n-D  BreakpointsForDimension1=da  BreakpointsForDimension2=Alpha  Table=Cnde  InternalRulePriority=Speed  RndMeth=Simplest
      settings: InputPortMap=u0,u1
  2-D Lookup Table3 : Lookup_n-D  BreakpointsForDimension1=dr  BreakpointsForDimension2=Beta  Table=Cndr  InternalRulePriority=Speed  RndMeth=Simplest
      settings: InputPortMap=u0,u1
  Add : Sum
  Add1 : Sum
  Add2 : Sum
  Add3 : Sum  Inputs=10
  Bus Selector : BusSelector  OutputSignals=q_dyn
  Bus Selector1 : BusSelector  OutputSignals=V_TAS
  Bus Selector2 : BusSelector  OutputSignals=alpha_beta_alpha_dot
  Bus Selector3 : BusSelector  OutputSignals=v_body
  Bus Selector4 : BusSelector  OutputSignals=Wind_Linear_Body,Wind_Angular_Body
  Bus Selector5 : BusSelector  OutputSignals=pqr,da_de_dr
  Constant10 : Constant  Value=chord
  Constant11 : Constant  Value=S
  Constant12 : Constant  Value=0
  Constant14 : Constant  Value=wing_span
  Constant8 : Constant  Value=Cn_alpha_dot
  Constant9 : Constant  Value=Cn_u
  Demux : Demux  Outputs=3
  Demux1 : Demux  Outputs=3
  Gain : Gain  Gain=2
  Gain1 : Gain  Gain=eps
  Gain2 : Gain  Gain=2
  Gain3 : Gain  Gain=eps
  Gain4 : Gain  Gain=2
  Gain5 : Gain  Gain=eps
  IsZero : simulink/Logic and Bit Operations/Compare To Zero  relop===  OutDataTypeStr=uint8
      settings: LibrarySourceBlock=|
      | simulink/Quick Insert/Logic and Bit
      | Operations/IsZero
  IsZero1 : simulink/Logic and Bit Operations/Compare To Zero  relop===  OutDataTypeStr=uint8
      settings: LibrarySourceBlock=|
      | simulink/Quick Insert/Logic and Bit
      | Operations/IsZero
  IsZero2 : simulink/Logic and Bit Operations/Compare To Zero  relop===  OutDataTypeStr=uint8
      settings: LibrarySourceBlock=|
      | simulink/Quick Insert/Logic and Bit
      | Operations/IsZero
  Product : Product  Inputs=**/
  Product{1,3,5,11..12} (5 alike) : Product
  Product10 : Product  Inputs=4
  Product2 : Product  Inputs=**/
  Product4 : Product  Inputs=**/
  Selector : Selector  InputPortWidth=3  IndexOptions=Index vector (dialog)  Indices=1  OutputSizes=1
  Selector1 : Selector  InputPortWidth=3  IndexOptions=Index vector (dialog)  Indices=3  OutputSizes=1
  Selector2 : Selector  InputPortWidth=3  IndexOptions=Index vector (dialog)  Indices=1  OutputSizes=1
  Selector3 : Selector  InputPortWidth=3  IndexOptions=Index vector (dialog)  Indices=2  OutputSizes=1
  Sum : Sum  Inputs=|+-
  Sum1 : Sum  Inputs=-+|
  Aero_Yaw_Moment : Outport  Unit=N*m
  wires:
  Constant14/1 -> [wing_span]
  [beta] -> 2-D Lookup Table3/2
  [dr] -> 2-D Lookup Table3/1
  [alpha] -> 2-D Lookup Table2/2
  [da] -> 2-D Lookup Table1/1
  [alpha] -> 2-D Lookup Table1/2
  [alpha] -> 1-D Lookup Table2/1
  1-D Lookup Table2/1 -> Product4/1
  [alpha] -> 1-D Lookup Table1/1
  1-D Lookup Table1/1 -> Product2/1
  [alpha] -> 1-D Lookup Table/1
  1-D Lookup Table/1 -> Product/1
  [beta] -> 2-D Lookup Table/2
  [alpha] -> 2-D Lookup Table/1
  Selector3/1 -> [beta]
  Bus Selector5/2 -> Demux1/1  "<da_de_dr>"
  Bus Selector5/1 -> Sum1/2  "<pqr>"
  [Aircraft_States] -> Bus Selector5/1
  Bus Selector4/2 -> Sum1/1  "<Wind_Angular_Body>"
  Sum1/1 -> Demux/1
  Sum/1 -> Selector2/1
  Bus Selector3/1 -> Sum/1  "<v_body>"
  Bus Selector4/1 -> Sum/2  "<Wind_Linear_Body>"
  [Wind_States] -> Bus Selector4/1
  Selector2/1 -> [u]
  Selector1/1 -> [alpha_dot]
  Selector/1 -> [alpha]
  Bus Selector2/1 -> Selector/1, Selector1/1, Selector3/1  "<alpha_beta_alpha_dot>"
  Bus Selector1/1 -> [V_TAS]  "<V_TAS>"
  Bus Selector/1 -> [q_dyn]  "<q_dyn>"
  [Aircraft_States] -> Bus Selector2/1, Bus Selector1/1, Bus Selector/1, Bus Selector3/1
  Wind_States/1 -> [Wind_States]
  Aircraft_States/1 -> [Aircraft_States]
  Demux1/3 -> [dr]
  2-D Lookup Table2/1 -> Add3/7
  [S] -> Product10/4
  Gain1/1 -> Add/2
  [V_TAS] -> IsZero2/1, Gain4/1
  [V_TAS] -> IsZero/1, Gain/1
  Add2/1 -> Product4/3
  Add/1 -> Product/3
  Constant12/1 -> Add3/1
  Product2/1 -> Product3/1
  [wing_span] -> Product10/2
  Add1/1 -> Product2/3
  Gain5/1 -> Add2/2
  Product4/1 -> Product5/1
  2-D Lookup Table1/1 -> Add3/6
  [q] -> Product3/2
  Add3/1 -> Product10/1
  Demux/3 -> [r]
  [V_TAS] -> Gain2/1, IsZero1/1
  Product5/1 -> Add3/5
  Gain/1 -> Add/1
  Gain4/1 -> Add2/1
  Gain3/1 -> Add1/2
  IsZero2/1 -> Gain5/1
  Gain2/1 -> Add1/1
  [q_dyn] -> Product10/3
  Demux1/1 -> [da]
  [chord] -> Product2/2
  IsZero1/1 -> Gain3/1
  [r] -> Product5/2
  [wing_span] -> Product/2
  Product/1 -> Product1/1
  Product1/1 -> Add3/3
  [p] -> Product1/2
  IsZero/1 -> Gain1/1
  2-D Lookup Table/1 -> Add3/2
  [wing_span] -> Product4/2
  Product3/1 -> Add3/4
  [de] -> 2-D Lookup Table2/1
  2-D Lookup Table3/1 -> Add3/8
  Demux/2 -> [q]
  Demux1/2 -> [de]
  Demux/1 -> [p]
  Product10/1 -> Aero_Yaw_Moment/1
  Constant10/1 -> [chord]
  Constant8/1 -> [CL_alpha_dot]
  Constant9/1 -> [CL_u]
  Constant11/1 -> [S]
  Product11/1 -> Add3/9
  [CL_alpha_dot] -> Product11/1
  Product12/1 -> Add3/10
  [CL_u] -> Product12/1
  [alpha_dot] -> Product11/2
  [u] -> Product12/2

== system Fixed_Wing_Model/Atmosphere_Model/Dynamic_Pressure ==
  rho : Inport  Unit=kg/m^3
  TAS : Inport  Port=2  Unit=m/s
  Gain : Gain  Gain=1/2
  Product : Product
  Square : Math  Operator=square
  q_dyn : Outport  Unit=N/m^2
  wires:
  Gain/1 -> q_dyn/1
  Product/1 -> Gain/1
  rho/1 -> Product/1
  TAS/1 -> Square/1
  Square/1 -> Product/2

== system Fixed_Wing_Model/Visualization/SkyHogg Rotation ==
  euler : Inport
  Constant : Constant  Value=zeros(9,3)
  Ppsi : Constant  Value=0
  Ptheta : Constant  Value=0
  Ramp : simulink/Sources/Ramp  slope=157  start=0  InitialOutput=0
  Reshape1 : Reshape  OutputDimensionality=Row vector (2-D)
  Reshape2 : Reshape  OutputDimensionality=Row vector (2-D)
  Vector Concatenate1 : Concatenate  Mode=Multidimensional array
  Vector Concatenate2 : Concatenate  Mode=Multidimensional array
  Vector Concatenate3 : Concatenate  NumInputs=3
  Rotation : Outport
  wires:
  euler/1 -> Reshape1/1  "Body"
  Vector Concatenate1/1 -> Rotation/1
  Constant/1 -> Vector Concatenate1/2
  Reshape1/1 -> Vector Concatenate2/1
  Vector Concatenate3/1 -> Reshape2/1  "Propeller"
  Ppsi/1 -> Vector Concatenate3/3  "psi"
  Ptheta/1 -> Vector Concatenate3/2  "theta"
  Ramp/1 -> Vector Concatenate3/1  "phi"
  Reshape2/1 -> Vector Concatenate2/2
  Vector Concatenate2/1 -> Vector Concatenate1/1

== system Fixed_Wing_Model/Visualization/SkyHogg Translation ==
  trans : Inport
  Constant : Constant  Value=zeros(10,3)
  Reshape : Reshape  OutputDimensionality=Row vector (2-D)
  Vector Concatenate : Concatenate  Mode=Multidimensional array
  Translation : Outport
  wires:
  Constant/1 -> Vector Concatenate/2
  Reshape/1 -> Vector Concatenate/1
  Vector Concatenate/1 -> Translation/1
  trans/1 -> Reshape/1
